simulink model "clik_inver"  (R2024a)
settings: Solver=ode45  StartTime=0.0  StopTime=45  RelTol=1e-3
model workspace (MAT data in the model file):
  x0 = 0
undefined symbols (not defined in the file or in its folder): DiscIntNeverNeededParam
settings Model: Creator=Peppe  LastModifiedBy=UTENTE
settings SolverCC: AlgebraicLoopSolver=TrustRegion
settings DebuggingCC: UnconnectedInputMsg=warning  UnconnectedOutputMsg=warning  UnconnectedLineMsg=warning
settings ModelReferenceCC: EnableRefExpFcnMdlSchedulingChecks=on
settings SFSimCC: CustomCodeUndefinedFunction=UseInterfaceOnly
settings RTWCC: GPUComputeCapability=3.5

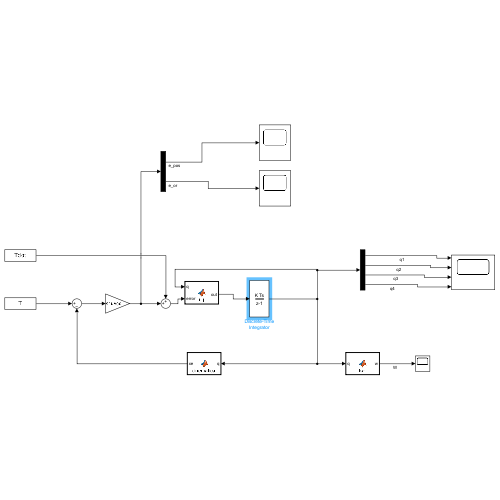
[thumbnail: Simulink's stored preview of the top-level diagram]
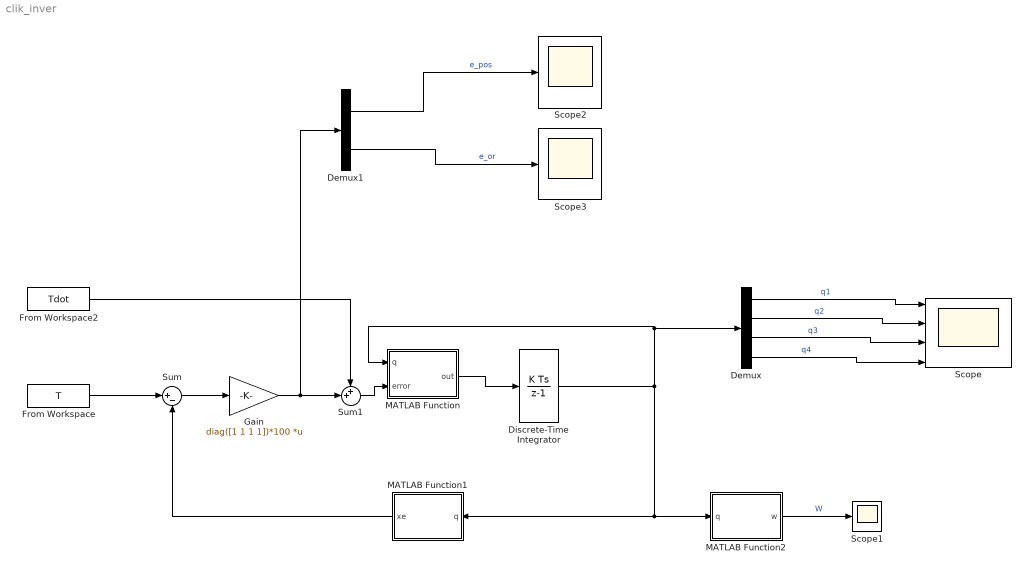
== system clik_inver ==
  Demux : Demux
  Demux1 : Demux  Outputs=2
  Discrete-Time Integrator : DiscreteIntegrator  InitialCondition=[-0.2505, 0.6750, 0, 0.5]'  SampleTime=0.001  ICPrevOutput=DiscIntNeverNeededParam  ICPrevScaledInput=DiscIntNeverNeededParam
  From Workspace : FromWorkspace  VariableName=T  SampleTime=0.001
  From Workspace2 : FromWorkspace  VariableName=Tdot  SampleTime=0.001
  Gain : Gain  Gain=diag([1 1 1 1])*100  Multiplication=Matrix(K*u) (u vector)
  MATLAB Function : MATLAB Function  TreatAsAtomicUnit=on
  MATLAB Function1 : MATLAB Function  TreatAsAtomicUnit=on
  MATLAB Function2 : MATLAB Function  TreatAsAtomicUnit=on
  Scope : Scope  NumInputPorts=4
  Scope1 : Scope
  Scope2 : Scope
  Scope3 : Scope
  Sum : Sum  Inputs=|+-
  Sum1 : Sum  Inputs=++|
  wires:
  From Workspace/1 -> Sum/1
  Discrete-Time Integrator/1 -> Demux/1, MATLAB Function/1(q), MATLAB Function2/1(q), MATLAB Function1/1(q)
  Sum/1 -> Gain/1
  MATLAB Function/1(out) -> Discrete-Time Integrator/1
  Sum1/1 -> MATLAB Function/2(error)
  From Workspace2/1 -> Sum1/1
  MATLAB Function1/1(xe) -> Sum/2
  Gain/1 -> Demux1/1, Sum1/2
  MATLAB Function2/1(w) -> Scope1/1  "W"
  Demux/1 -> Scope/1  "q1"
  Demux/2 -> Scope/2  "q2"
  Demux/3 -> Scope/3  "q3"
  Demux/4 -> Scope/4  "q4"
  Demux1/1 -> Scope2/1  "e_pos"
  Demux1/2 -> Scope3/1  "e_or"

== matlab function clik_inver/MATLAB Function ==
  data: q input; out output; error input
function out= i_j(q,error)

J=[-0.5*sin(q(1))-0.5*sin(q(1)+q(2)) -0.5*sin(q(1)+q(2)) 0 0;
    0.5*cos(q(1))+0.5*cos(q(1)+q(2)) 0.5*cos(q(1)+q(2)) 0 0;
    0 0 -1 0;
    1 1 0 -1];

J_t=inv(J);

%  trans_Jacobian=J_t;
 out = J_t * error;
end

== matlab function clik_inver/MATLAB Function2 ==
  data: q input; w output
function w = fcn(q)
a1 = 0.5;
a2 = 0.5;
w =(sin(q(1) + q(2))*cos(q(1)))/4 - (cos(q(1) + q(2))*sin(q(1)))/4;
end

== matlab function clik_inver/MATLAB Function1 ==
  data: q input; xe output
function xe = cinematica(q)
xe_=[0.5*cos(q(1))+0.5*cos(q(1)+q(2));
    0.5*sin(q(1))+0.5*sin(q(1)+q(2));
        1-q(3);
        q(1)+q(2)-q(4)];
xe = xe_;
